simulink subsystem "PipelinedAccumulator"  (R2024a)
settings: Solver=VariableStepAuto  StartTime=0.0  StopTime=10.0  RelTol=1e-3
model mask{PipelineLength=0}
libraries: hdlsllib x2
settings Model: Creator=versal  LastModifiedBy=versal

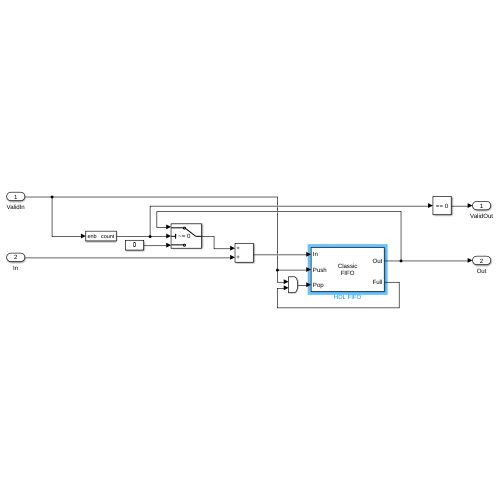
[thumbnail: Simulink's stored preview of the top-level diagram]
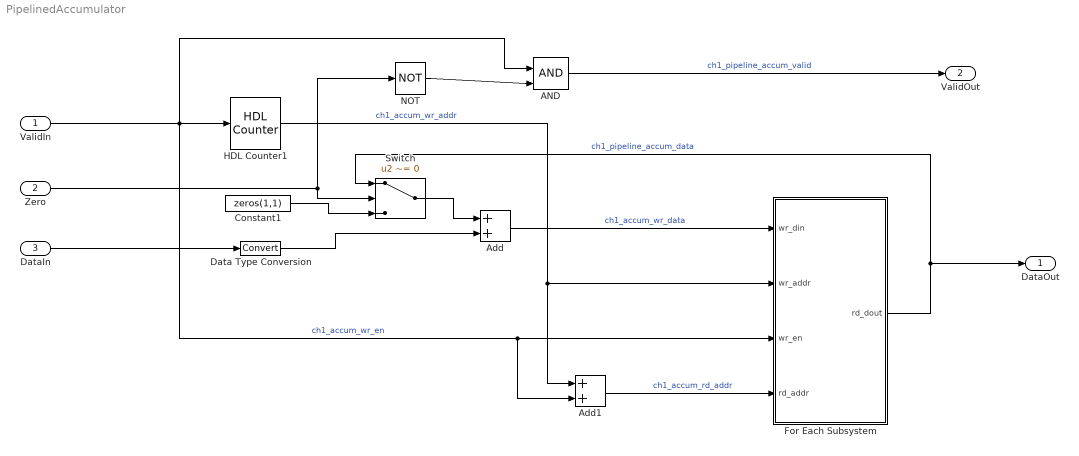
== system PipelinedAccumulator ==
  ValidIn : Inport
  Zero : Inport  Port=2
  DataIn : Inport  Port=3
  AND : Logic  IconShape=distinctive  AllPortsSameDT=off  OutDataTypeStr=boolean
  Add : Sum  OutDataTypeStr=Inherit: Same as accumulator  AccumDataTypeStr=fixdt(1,48,6)  InputSameDT=on  SaturateOnIntegerOverflow=on  LockScale=on
  Add1 : Sum  OutDataTypeStr=Inherit: Same as first input
  Constant1 : Constant  Value=zeros(1,1)  VectorParams1D=off  OutDataTypeStr=Inherit: Inherit via back propagation  LockScale=on
  Data Type Conversion : DataTypeConversion  SaturateOnIntegerOverflow=off  RndMeth=Floor
  For Each Subsystem : Subsystem  TreatAsAtomicUnit=on
      settings: MinAlgLoopOccurrences=on
  HDL Counter1 : hdlsllib/Sources/HDL Counter  CountType=Count limited  CountInit=0  CountStep=1  CountMax=PipelineLength-1  CountFromType=Initial value  CountFrom=0  CountResetPort=off  CountLoadPort=off  CountEnbPort=on  CountDirPort=off  CountHitOutputPort=off  CountDataType=Unsigned  CountWordLen=6  CountFracLen=0  CountSampTime=1
  NOT : Logic  Operator=NOT  IconShape=distinctive  AllPortsSameDT=off  OutDataTypeStr=boolean
  Switch : Switch  Criteria=u2 ~= 0  SaturateOnIntegerOverflow=off  InputSameDT=off  OutDataTypeStr=Inherit: Same as first input
  DataOut : Outport
  ValidOut : Outport  Port=2
  wires:
  Data Type Conversion/1 -> Add/2
  AND/1 -> ValidOut/1  "ch1_pipeline_accum_valid"
  Zero/1 -> NOT/1, Switch/2
  NOT/1 -> AND/2
  Add1/1 -> For Each Subsystem/4(rd_addr)  "ch1_accum_rd_addr"
  DataIn/1 -> Data Type Conversion/1
  Switch/1 -> Add/1
  HDL Counter1/1 -> For Each Subsystem/2(wr_addr), Add1/1  "ch1_accum_wr_addr"
  Constant1/1 -> Switch/3
  Add/1 -> For Each Subsystem/1(wr_din)  "ch1_accum_wr_data"
  For Each Subsystem/1(rd_dout) -> DataOut/1, Switch/1  "ch1_pipeline_accum_data"
  ValidIn/1 -> AND/1, For Each Subsystem/3(wr_en), Add1/2, HDL Counter1/1  "ch1_accum_wr_en"

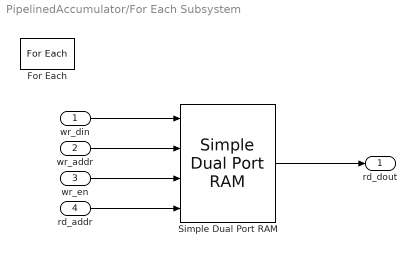
== system PipelinedAccumulator/For Each Subsystem ==
  wr_din : Inport  Partition=on  PartitionDimension=1  PartitionWidth=1  PartitionOffset=0
  wr_addr : Inport  Port=2
  wr_en : Inport  Port=3
  rd_addr : Inport  Port=4
  For Each : ForEach  DisableCoverage=on
  Simple Dual Port RAM : hdlsllib/HDL RAMs/Simple Dual Port RAM  ram_size=log2(PipelineLength)
  rd_dout : Outport  ConcatenationDimension=1
  wires:
  wr_en/1 -> Simple Dual Port RAM/3
  Simple Dual Port RAM/1 -> rd_dout/1
  wr_addr/1 -> Simple Dual Port RAM/2
  wr_din/1 -> Simple Dual Port RAM/1
  rd_addr/1 -> Simple Dual Port RAM/4
